simulink model "sl_closed_loop_2"  (R2020a)
settings: Solver=ode45  StartTime=0.0  StopTime=3  MaxStep=0.01  RelTol=1e-5  EnableMultiTasking=on
values from neighbouring files (symbols this model uses):
  A = zeros(4,4)    [closed_loop_1.m]    (also in closed_loop_2.m; open_loop.m)
  A2 = zeros(4,4)    [closed_loop_2.m]
  B = zeros(4,1)    [closed_loop_1.m]    (also in closed_loop_2.m; open_loop.m)
  B2 = zeros(4,2)    [closed_loop_2.m]
  C = eye(4)    [closed_loop_1.m]    (also in closed_loop_2.m = [1 0 0 0; open_loop.m = [1 0 0 0)
  C2 = zeros(2,4)    [closed_loop_2.m]
  D = zeros(4,1)    [closed_loop_1.m]    (also in closed_loop_2.m = [0; open_loop.m = zeros(2,1))
  D2 = zeros(2,2)    [closed_loop_2.m]
  K = K(1,:)    [closed_loop_1.m]    (also in closed_loop_2.m)
  T_s = 0.005    [closed_loop_2.m]
  x0 = [0  10*pi/180 0 0 ]    [closed_loop_1.m]    (also in closed_loop_2.m)
  x_d = [0.1 0 0 0]    [closed_loop_1.m]    (also in closed_loop_2.m)
settings Model: Creator=magudelo  LastModifiedBy=LouisDecloedt
settings DataIOCC: LimitDataPoints=on  SaveFormat=Array  SignalLoggingSaveFormat=ModelDataLogs  ReturnWorkspaceOutputs=off
settings OptimizationCC: ExpressionDepthLimit=2147483647  LifeSpan=inf
settings DebuggingCC: UnderspecifiedInitializationDetection=Classic  MergeDetectMultiDrivingBlocksExec=none  SolverPrmCheckMsg=warning  FcnCallInpInsideContextMsg=warning  AllowSymbolicDim=off  StateNameClashWarn=warning  SFUnexpectedBacktrackingDiag=warning  SFNoUnconditionalDefaultTransitionDiag=warning  SFExecutionAtInitializationDiag=none  ArithmeticOperatorsInVariantConditions=warning
settings HardwareCC: ProdBitPerPointer=32  ProdBitPerSizeT=32  ProdBitPerPtrDiffT=32  ProdLargestAtomicFloat=None  ProdIntDivRoundTo=Undefined  ProdEndianess=Unspecified  ProdWordSize=32  ProdHWDeviceType=32-bit Generic
settings ModelReferenceCC: PropagateSignalLabelsOutOfModel=off
settings SFSimCC: SimUseLocalCustomCode=off  CustomCodeUndefinedFunction=UseInterfaceOnly
settings RTWCC: RTWUseLocalCustomCode=off
settings CodeAppCC: StateflowObjectComments=on
settings GRTTargetCC: TargetLangStandard=C89/C90 (ANSI)  CombineOutputUpdateFcns=off  GRTInterface=on
settings ConfigComp: CovMetricSettings=dw  CovHtmlReporting=on  CovSaveCumulativeToWorkspaceVar=on  CovSaveSingleToWorkspaceVar=on  CovExternalEMLEnable=off

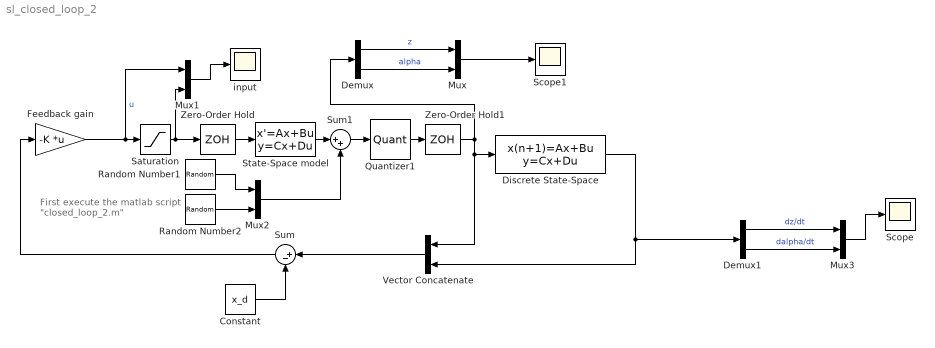
== system sl_closed_loop_2 ==
  note: First execute the matlab
      |  script "closed_loop_2.m"
  Constant : Constant  Value=x_d
  Demux : Demux  Outputs=2
  Demux1 : Demux  Outputs=2
  Discrete State-Space : DiscreteStateSpace  A=A2  B=B2  C=C2  D=D2  InitialCondition=[0 0 0 0]  SampleTime=-1
  Feedback gain : Gain  Tag=Feedback gain  Description=f  Gain=-K  Multiplication=Matrix(K*u)
  Mux{,1..3} (4 alike) : Mux  Inputs=2
  Quantizer1 : Quantizer  QuantizationInterval=1/(2^16)
  Random Number1 : RandomNumber  Variance=1e-7  SampleTime=T_s
  Random Number2 : RandomNumber  Variance=1e-7  SampleTime=T_s
  Saturation : Saturate  UpperLimit=5  LowerLimit=-5
  Scope : Scope
  Scope1 : Scope
  State-Space model : StateSpace  A=A  B=B  C=C  D=D  InitialCondition=x0
  Sum : Sum  Inputs=|+-
  Sum1 : Sum  Inputs=|++
  Vector Concatenate : Concatenate
  Zero-Order Hold : ZeroOrderHold  SampleTime=-1
  Zero-Order Hold1 : ZeroOrderHold  SampleTime=T_s
  input : Scope
  wires:
  Mux1/1 -> input/1
  Saturation/1 -> Mux1/2, Zero-Order Hold/1
  Zero-Order Hold/1 -> State-Space model/1
  Quantizer1/1 -> Zero-Order Hold1/1
  Discrete State-Space/1 -> Demux1/1, Vector Concatenate/2
  Feedback gain/1 -> Mux1/1, Saturation/1  "u"
  Constant/1 -> Sum/2
  Sum/1 -> Feedback gain/1
  Vector Concatenate/1 -> Sum/1
  Zero-Order Hold1/1 -> Vector Concatenate/1, Discrete State-Space/1, Demux/1
  Demux/1 -> Mux/1  "z"
  Random Number2/1 -> Mux2/2
  Random Number1/1 -> Mux2/1
  Mux2/1 -> Sum1/2
  State-Space model/1 -> Sum1/1
  Sum1/1 -> Quantizer1/1
  Demux/2 -> Mux/2  "alpha"
  Mux/1 -> Scope1/1
  Demux1/1 -> Mux3/1  "dz/dt"
  Demux1/2 -> Mux3/2  "dalpha/dt"
  Mux3/1 -> Scope/1
